simulink model "a4"  (R2018b)
settings: Solver=ode23tb  StartTime=0.0  StopTime=24*60*60  MaxStep=60  RelTol=1e-4
PreLoadFcn:
  | load('solar_load_data_24h.mat')
(part 1 of 2)
settings Model: Creator=alavi  LastModifiedBy=alavi
settings SolverCC: InitialStep=1e-4
settings SFSimCC: SimUseLocalCustomCode=off
settings RTWCC: RTWUseLocalCustomCode=off
settings CodeAppCC: StateflowObjectComments=on

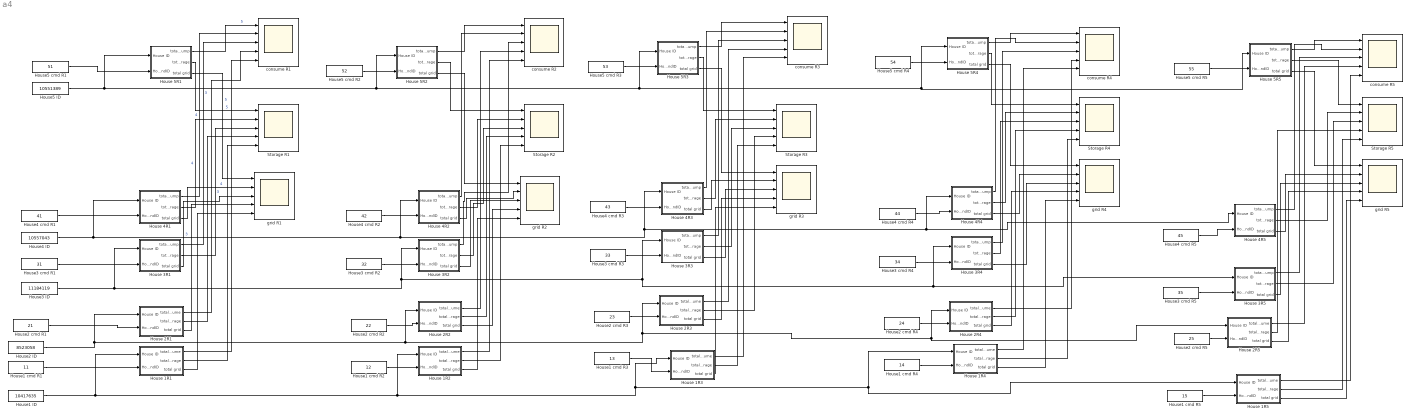
== system a4 ==
  House 1R1 : Subsystem
  House 1R2 : Subsystem
  House 1R3 : Subsystem
  House 1R4 : Subsystem
  House 1R5 : Subsystem
  House 2R1 : Subsystem
  House 2R2 : Subsystem
  House 2R3 : Subsystem
  House 2R4 : Subsystem
  House 2R5 : Subsystem
  House 3R1 : Subsystem
  House 3R2 : Subsystem
  House 3R3 : Subsystem
  House 3R4 : Subsystem
  House 3R5 : Subsystem
  House 4R1 : Subsystem
  House 4R2 : Subsystem
  House 4R3 : Subsystem
  House 4R4 : Subsystem
  House 4R5 : Subsystem
  House 5R1 : Subsystem
  House 5R2 : Subsystem
  House 5R3 : Subsystem
  House 5R4 : Subsystem
  House 5R5 : Subsystem
  House1 ID : Constant  Value=10417635
  House1 cmd R1 : Constant  Value=11
  House1 cmd R2 : Constant  Value=12
  House1 cmd R3 : Constant  Value=13
  House1 cmd R4 : Constant  Value=14
  House1 cmd R5 : Constant  Value=15
  House2 ID : Constant  Value=8523058
  House2 cmd R1 : Constant  Value=21
  House2 cmd R2 : Constant  Value=22
  House2 cmd R3 : Constant  Value=23
  House2 cmd R4 : Constant  Value=24
  House2 cmd R5 : Constant  Value=25
  House3 ID : Constant  Value=11184119
  House3 cmd R1 : Constant  Value=31
  House3 cmd R2 : Constant  Value=32
  House3 cmd R3 : Constant  Value=33
  House3 cmd R4 : Constant  Value=34
  House3 cmd R5 : Constant  Value=35
  House4 ID : Constant  Value=10557043
  House4 cmd R1 : Constant  Value=41
  House4 cmd R2 : Constant  Value=42
  House4 cmd R3 : Constant  Value=43
  House4 cmd R4 : Constant  Value=44
  House4 cmd R5 : Constant  Value=45
  House5 ID : Constant  Value=10551389
  House5 cmd R1 : Constant  Value=51
  House5 cmd R2 : Constant  Value=52
  House5 cmd R3 : Constant  Value=53
  House5 cmd R4 : Constant  Value=54
  House5 cmd R5 : Constant  Value=55
  "Storage R1 " : Scope  NumInputPorts=5
  Storage R{2..5} (4 alike) : Scope  NumInputPorts=5
  "consume R1 " : Scope  NumInputPorts=5
  consume R{2..5} (4 alike) : Scope  NumInputPorts=5
  "grid R1 " : Scope  NumInputPorts=5
  grid R{2..5} (4 alike) : Scope  NumInputPorts=5
  wires:
  House1 cmd R1/1 -> House 1R1/2(House CommandID)
  House2 cmd R1/1 -> House 2R1/2(House CommandID)
  House3 cmd R1/1 -> House 3R1/2(House CommandID)
  House4 cmd R1/1 -> House 4R1/2(House CommandID)
  House1 cmd R2/1 -> House 1R2/2(House CommandID)
  House2 cmd R2/1 -> House 2R2/2(House CommandID)
  House1 cmd R3/1 -> House 1R3/2(House CommandID)
  House2 cmd R3/1 -> House 2R3/2(House CommandID)
  House1 cmd R4/1 -> House 1R4/2(House CommandID)
  House2 cmd R4/1 -> House 2R4/2(House CommandID)
  House1 ID/1 -> House 1R2/1(House ID), House 1R3/1(House ID), House 1R5/1(House ID), House 1R4/1(House ID), House 1R1/1(House ID)
  House1 cmd R5/1 -> House 1R5/2(House CommandID)
  House4 cmd R2/1 -> House 4R2/2(House CommandID)
  House3 cmd R2/1 -> House 3R2/2(House CommandID)
  House4 cmd R3/1 -> House 4R3/2(House CommandID)
  House3 cmd R3/1 -> House 3R3/2(House CommandID)
  House4 cmd R4/1 -> House 4R4/2(House CommandID)
  House3 cmd R4/1 -> House 3R4/2(House CommandID)
  House4 cmd R5/1 -> House 4R5/2(House CommandID)
  House4 ID/1 -> House 4R1/1(House ID), House 4R2/1(House ID), House 4R3/1(House ID), House 4R5/1(House ID), House 4R4/1(House ID)
  House3 ID/1 -> House 3R1/1(House ID), House 3R2/1(House ID), House 3R3/1(House ID), House 3R5/1(House ID), House 3R4/1(House ID)
  House3 cmd R5/1 -> House 3R5/2(House CommandID)
  House5 cmd R2/1 -> House 5R2/2(House CommandID)
  House5 cmd R1/1 -> House 5R1/2(House CommandID)
  House5 ID/1 -> House 5R2/1(House ID), House 5R3/1(House ID), House 5R5/1(House ID), House 5R4/1(House ID), House 5R1/1(House ID)
  House5 cmd R3/1 -> House 5R3/2(House CommandID)
  House5 cmd R4/1 -> House 5R4/2(House CommandID)
  House5 cmd R5/1 -> House 5R5/2(House CommandID)
  House2 ID/1 -> House 2R2/1(House ID), House 2R3/1(House ID), House 2R5/1(House ID), House 2R4/1(House ID), House 2R1/1(House ID)
  House 5R1/1(total consump) -> "consume R1 "/1  "5"
  House 5R1/2(total storage) -> "Storage R1 "/1  "5"
  House 5R1/3(total grid) -> "grid R1 "/1  "5"
  House 5R2/1(total consump) -> consume R2/1
  House 5R2/2(total storage) -> Storage R2/1
  House 5R2/3(total grid) -> grid R2/1
  House 5R3/1(total consump) -> consume R3/1
  House 5R3/2(total storage) -> Storage R3/1
  House 5R3/3(total grid) -> grid R3/1
  House 5R4/1(total consump) -> consume R4/1
  House 5R4/2(total storage) -> Storage R4/1
  House 5R4/3(total grid) -> grid R4/1
  House 5R5/1(total consump) -> consume R5/1
  House 5R5/2(total storage) -> Storage R5/1
  House 5R5/3(total grid) -> grid R5/1
  House 4R1/1(total consump) -> "consume R1 "/2  "4"
  House 4R1/2(total storage) -> "Storage R1 "/2  "4"
  House 4R1/3(total grid) -> "grid R1 "/2  "4"
  House 3R1/1(total consump) -> "consume R1 "/3  "3"
  House 3R1/2(total storage) -> "Storage R1 "/3  "3"
  House 3R1/3(total grid) -> "grid R1 "/3  "3"
  House 4R2/1(total consump) -> consume R2/2
  House 4R2/2(total storage) -> Storage R2/2
  House 4R2/3(total grid) -> grid R2/2
  House 3R2/1(total consump) -> consume R2/3
  House 3R2/2(total storage) -> Storage R2/3
  House 3R2/3(total grid) -> grid R2/3
  House 4R3/1(total consump) -> consume R3/2
  House 4R3/2(total storage) -> Storage R3/2
  House 4R3/3(total grid) -> grid R3/2
  House 3R3/1(total consump) -> consume R3/3
  House 3R3/2(total storage) -> Storage R3/3
  House 3R3/3(total grid) -> grid R3/3
  House 4R4/1(total consump) -> consume R4/2
  House 4R4/2(total storage) -> Storage R4/2
  House 4R4/3(total grid) -> grid R4/2
  House 3R4/1(total consump) -> consume R4/3
  House 3R4/2(total storage) -> Storage R4/3
  House 3R4/3(total grid) -> grid R4/3
  House 4R5/1(total consump) -> consume R5/2
  House 4R5/2(total storage) -> Storage R5/2
  House 3R5/1(total consump) -> consume R5/3
  House 4R5/3(total grid) -> grid R5/2
  House 3R5/2(total storage) -> Storage R5/3
  House 3R5/3(total grid) -> grid R5/3
  House 2R1/1(total consume) -> "consume R1 "/4
  House 2R1/2(total storage) -> "Storage R1 "/4
  House 2R1/3(total grid) -> "grid R1 "/4
  House 2R2/1(total consume) -> consume R2/4
  House 2R2/2(total storage) -> Storage R2/4
  House 2R2/3(total grid) -> grid R2/4
  House 2R3/1(total consume) -> consume R3/4
  House 2R3/2(total storage) -> Storage R3/4
  House 2R3/3(total grid) -> grid R3/4
  House 2R4/1(total consume) -> consume R4/4
  House 2R4/2(total storage) -> Storage R4/4
  House 2R4/3(total grid) -> grid R4/4
  House 2R5/1(total consume) -> consume R5/4
  House 2R5/2(total storage) -> Storage R5/4
  House 2R5/3(total grid) -> grid R5/4
  House 1R1/1(total consume) -> "consume R1 "/5
  House 1R1/2(total storage) -> "Storage R1 "/5
  House 1R1/3(total grid) -> "grid R1 "/5
  House 1R2/1(total consume) -> consume R2/5
  House 1R2/2(total storage) -> Storage R2/5
  House 1R2/3(total grid) -> grid R2/5
  House 1R3/1(total consume) -> consume R3/5
  House 1R3/2(total storage) -> Storage R3/5
  House 1R3/3(total grid) -> grid R3/5
  House 1R4/1(total consume) -> consume R4/5
  House 1R4/2(total storage) -> Storage R4/5
  House 1R4/3(total grid) -> grid R4/5
  House 1R5/1(total consume) -> consume R5/5
  House 1R5/2(total storage) -> Storage R5/5
  House 1R5/3(total grid) -> grid R5/5
  House2 cmd R5/1 -> House 2R5/2(House CommandID)

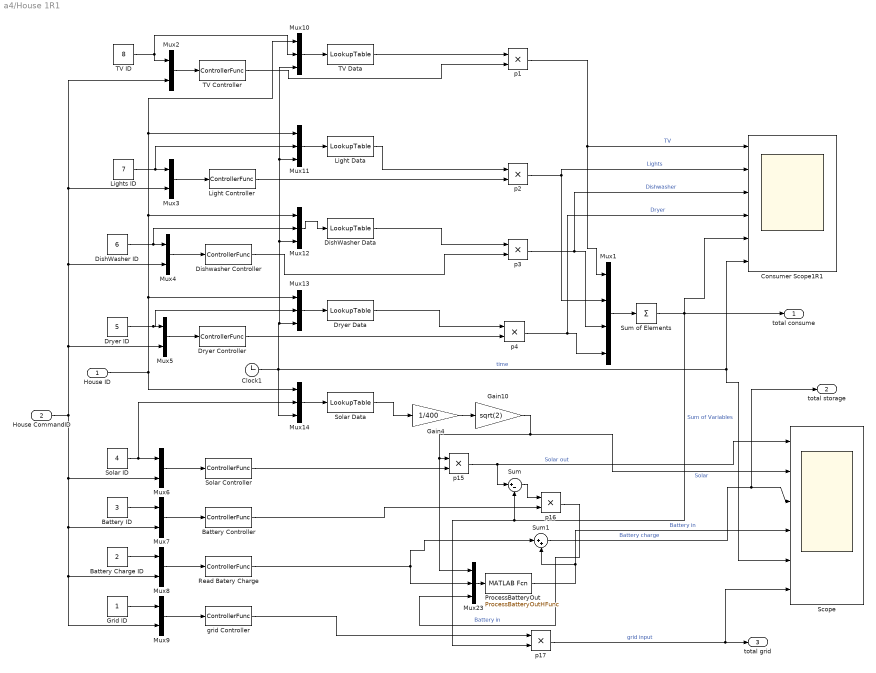
== system a4/House 1R1 ==
  House ID : Inport
  House CommandID : Inport  Port=2
  Battery Charge ID : Constant  Value=2
  Battery Controller : MATLABFcn  MATLABFcn=ControllerFunc  OutputSignalType=real
  Battery ID : Constant  Value=3
  Clock1 : Clock
  Consumer Scope1R1 : Scope  NumInputPorts=6
  DishWasher Data : MATLABFcn  MATLABFcn=LookupTable  OutputSignalType=real
  DishWasher ID : Constant  Value=6
  Dishwasher Controller : MATLABFcn  MATLABFcn=ControllerFunc  OutputSignalType=real
  Dryer Controller : MATLABFcn  MATLABFcn=ControllerFunc  OutputSignalType=real
  Dryer Data : MATLABFcn  MATLABFcn=LookupTable  OutputSignalType=real
  Dryer ID : Constant  Value=5
  Gain10 : Gain  Gain=sqrt(2)
  Gain4 : Gain  Gain=1/400
  Grid ID : Constant
  Light Controller : MATLABFcn  MATLABFcn=ControllerFunc  OutputSignalType=real
  Light Data : MATLABFcn  MATLABFcn=LookupTable  OutputSignalType=real
  Lights ID : Constant  Value=7
  Mux1 : Mux
  Mux{10..14,23} (6 alike) : Mux  Inputs=3
  Mux{2..9} (8 alike) : Mux  Inputs=2
  ProcessBatteryOut : MATLABFcn  MATLABFcn=ProcessBatteryOutHFunc  OutputSignalType=real
  Read Batery Charge : MATLABFcn  MATLABFcn=ControllerFunc  OutputSignalType=real
  Scope : Scope  NumInputPorts=6
  Solar Controller : MATLABFcn  MATLABFcn=ControllerFunc  OutputSignalType=real
  Solar Data : MATLABFcn  MATLABFcn=LookupTable  OutputSignalType=real
  Solar ID : Constant  Value=4
  Sum : Sum  Inputs=|+-
  Sum of Elements : Sum  Inputs=+
  Sum1 : Sum  Inputs=|++
  TV Controller : MATLABFcn  MATLABFcn=ControllerFunc  OutputSignalType=real
  TV Data : MATLABFcn  MATLABFcn=LookupTable  OutputSignalType=real
  TV ID : Constant  Value=8
  grid Controller : MATLABFcn  MATLABFcn=ControllerFunc  OutputSignalType=real
  p{1..4,15..17} (7 alike) : Product
  total consume : Outport
  total storage : Outport  Port=2
  total grid : Outport  Port=3
  wires:
  Clock1/1 -> Mux11/3, Mux10/3, Mux12/3, Mux13/3, Mux14/3, Scope/5, Consumer Scope1R1/6  "time"
  TV Data/1 -> p1/1
  Mux1/1 -> Sum of Elements/1
  p1/1 -> Consumer Scope1R1/1, Mux1/1  "TV"
  Sum of Elements/1 -> Consumer Scope1R1/5, total consume/1, p17/2, Sum/2  "Sum of Variables"
  p4/1 -> Consumer Scope1R1/4, Mux1/4  "Dryer"
  p2/1 -> Consumer Scope1R1/2, Mux1/2  "Lights"
  p3/1 -> Consumer Scope1R1/3, Mux1/3  "Dishwasher"
  Light Controller/1 -> p2/2
  Dishwasher Controller/1 -> p3/2
  Solar Data/1 -> Gain4/1
  Solar Controller/1 -> p15/2
  Gain10/1 -> Scope/2, Mux23/1, p15/1  "Solar"
  p15/1 -> Sum/1, Scope/1  "Solar out"
  Sum/1 -> p16/1
  Battery Controller/1 -> p16/2
  Sum1/1 -> total storage/1, Scope/3  "Battery charge"
  grid Controller/1 -> p17/1
  p17/1 -> Scope/6, total grid/1  "grid input"
  Read Batery Charge/1 -> Mux23/2, Sum1/1
  p16/1 -> Mux23/3  "Battery in"
  ProcessBatteryOut/1 -> Scope/4, Sum1/2  "Battery in"
  Light Data/1 -> p2/1
  DishWasher Data/1 -> p3/1
  Dryer Data/1 -> p4/1
  Dryer Controller/1 -> p4/2
  Gain4/1 -> Gain10/1
  TV ID/1 -> Mux2/1, Mux10/2
  House ID/1 -> Mux14/1, Mux10/1, Mux11/1, Mux12/1, Mux13/1
  Lights ID/1 -> Mux11/2, Mux3/1
  Mux3/1 -> Light Controller/1
  DishWasher ID/1 -> Mux12/2, Mux4/1
  Mux4/1 -> Dishwasher Controller/1
  Mux5/1 -> Dryer Controller/1
  Dryer ID/1 -> Mux13/2, Mux5/1
  Mux6/1 -> Solar Controller/1
  Solar ID/1 -> Mux14/2, Mux6/1
  Mux7/1 -> Battery Controller/1
  Mux8/1 -> Read Batery Charge/1
  Mux9/1 -> grid Controller/1
  Battery ID/1 -> Mux7/1
  Battery Charge ID/1 -> Mux8/1
  Grid ID/1 -> Mux9/1
  Mux10/1 -> TV Data/1
  Mux11/1 -> Light Data/1
  Mux12/1 -> DishWasher Data/1
  Mux13/1 -> Dryer Data/1
  Mux14/1 -> Solar Data/1
  TV Controller/1 -> p1/2
  Mux2/1 -> TV Controller/1
  House CommandID/1 -> Mux9/2, Mux8/2, Mux7/2, Mux6/2, Mux3/2, Mux2/2, Mux4/2, Mux5/2
  Mux23/1 -> ProcessBatteryOut/1

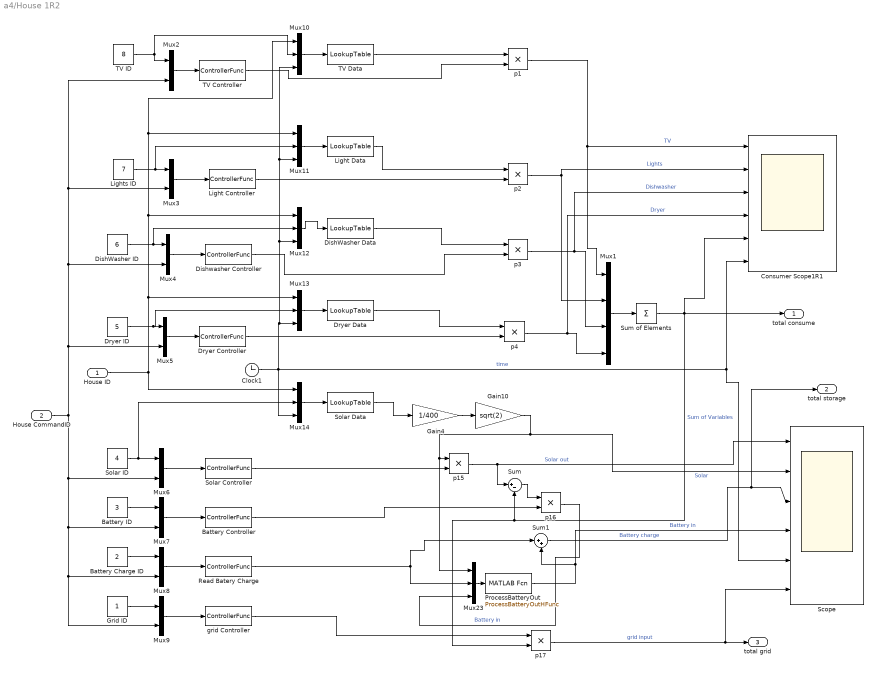
== system a4/House 1R2 ==
  House ID : Inport
  House CommandID : Inport  Port=2
  Battery Charge ID : Constant  Value=2
  Battery Controller : MATLABFcn  MATLABFcn=ControllerFunc  OutputSignalType=real
  Battery ID : Constant  Value=3
  Clock1 : Clock
  Consumer Scope1R1 : Scope  NumInputPorts=6
  DishWasher Data : MATLABFcn  MATLABFcn=LookupTable  OutputSignalType=real
  DishWasher ID : Constant  Value=6
  Dishwasher Controller : MATLABFcn  MATLABFcn=ControllerFunc  OutputSignalType=real
  Dryer Controller : MATLABFcn  MATLABFcn=ControllerFunc  OutputSignalType=real
  Dryer Data : MATLABFcn  MATLABFcn=LookupTable  OutputSignalType=real
  Dryer ID : Constant  Value=5
  Gain10 : Gain  Gain=sqrt(2)
  Gain4 : Gain  Gain=1/400
  Grid ID : Constant
  Light Controller : MATLABFcn  MATLABFcn=ControllerFunc  OutputSignalType=real
  Light Data : MATLABFcn  MATLABFcn=LookupTable  OutputSignalType=real
  Lights ID : Constant  Value=7
  Mux1 : Mux
  Mux{10..14,23} (6 alike) : Mux  Inputs=3
  Mux{2..9} (8 alike) : Mux  Inputs=2
  ProcessBatteryOut : MATLABFcn  MATLABFcn=ProcessBatteryOutHFunc  OutputSignalType=real
  Read Batery Charge : MATLABFcn  MATLABFcn=ControllerFunc  OutputSignalType=real
  Scope : Scope  NumInputPorts=6
  Solar Controller : MATLABFcn  MATLABFcn=ControllerFunc  OutputSignalType=real
  Solar Data : MATLABFcn  MATLABFcn=LookupTable  OutputSignalType=real
  Solar ID : Constant  Value=4
  Sum : Sum  Inputs=|+-
  Sum of Elements : Sum  Inputs=+
  Sum1 : Sum  Inputs=|++
  TV Controller : MATLABFcn  MATLABFcn=ControllerFunc  OutputSignalType=real
  TV Data : MATLABFcn  MATLABFcn=LookupTable  OutputSignalType=real
  TV ID : Constant  Value=8
  grid Controller : MATLABFcn  MATLABFcn=ControllerFunc  OutputSignalType=real
  p{1..4,15..17} (7 alike) : Product
  total consume : Outport
  total storage : Outport  Port=2
  total grid : Outport  Port=3
  wires:
  Mux23/1 -> ProcessBatteryOut/1
  House CommandID/1 -> Mux5/2, Mux4/2, Mux2/2, Mux3/2, Mux6/2, Mux7/2, Mux8/2, Mux9/2
  Mux2/1 -> TV Controller/1
  TV Controller/1 -> p1/2
  Mux14/1 -> Solar Data/1
  Mux13/1 -> Dryer Data/1
  Mux12/1 -> DishWasher Data/1
  Mux11/1 -> Light Data/1
  Mux10/1 -> TV Data/1
  Grid ID/1 -> Mux9/1
  Battery Charge ID/1 -> Mux8/1
  Battery ID/1 -> Mux7/1
  Mux9/1 -> grid Controller/1
  Mux8/1 -> Read Batery Charge/1
  Mux7/1 -> Battery Controller/1
  Solar ID/1 -> Mux6/1, Mux14/2
  Mux6/1 -> Solar Controller/1
  Dryer ID/1 -> Mux5/1, Mux13/2
  Mux5/1 -> Dryer Controller/1
  Mux4/1 -> Dishwasher Controller/1
  DishWasher ID/1 -> Mux4/1, Mux12/2
  Mux3/1 -> Light Controller/1
  Lights ID/1 -> Mux3/1, Mux11/2
  House ID/1 -> Mux13/1, Mux12/1, Mux11/1, Mux10/1, Mux14/1
  TV ID/1 -> Mux10/2, Mux2/1
  Gain4/1 -> Gain10/1
  Dryer Controller/1 -> p4/2
  Dryer Data/1 -> p4/1
  DishWasher Data/1 -> p3/1
  Light Data/1 -> p2/1
  ProcessBatteryOut/1 -> Sum1/2, Scope/4  "Battery in"
  p16/1 -> Mux23/3  "Battery in"
  Read Batery Charge/1 -> Sum1/1, Mux23/2
  p17/1 -> total grid/1, Scope/6  "grid input"
  grid Controller/1 -> p17/1
  Sum1/1 -> Scope/3, total storage/1  "Battery charge"
  Battery Controller/1 -> p16/2
  Sum/1 -> p16/1
  p15/1 -> Scope/1, Sum/1  "Solar out"
  Gain10/1 -> p15/1, Mux23/1, Scope/2  "Solar"
  Solar Controller/1 -> p15/2
  Solar Data/1 -> Gain4/1
  Dishwasher Controller/1 -> p3/2
  Light Controller/1 -> p2/2
  p3/1 -> Mux1/3, Consumer Scope1R1/3  "Dishwasher"
  p2/1 -> Mux1/2, Consumer Scope1R1/2  "Lights"
  p4/1 -> Mux1/4, Consumer Scope1R1/4  "Dryer"
  Sum of Elements/1 -> Sum/2, p17/2, total consume/1, Consumer Scope1R1/5  "Sum of Variables"
  p1/1 -> Mux1/1, Consumer Scope1R1/1  "TV"
  Mux1/1 -> Sum of Elements/1
  TV Data/1 -> p1/1
  Clock1/1 -> Consumer Scope1R1/6, Scope/5, Mux14/3, Mux13/3, Mux12/3, Mux10/3, Mux11/3  "time"

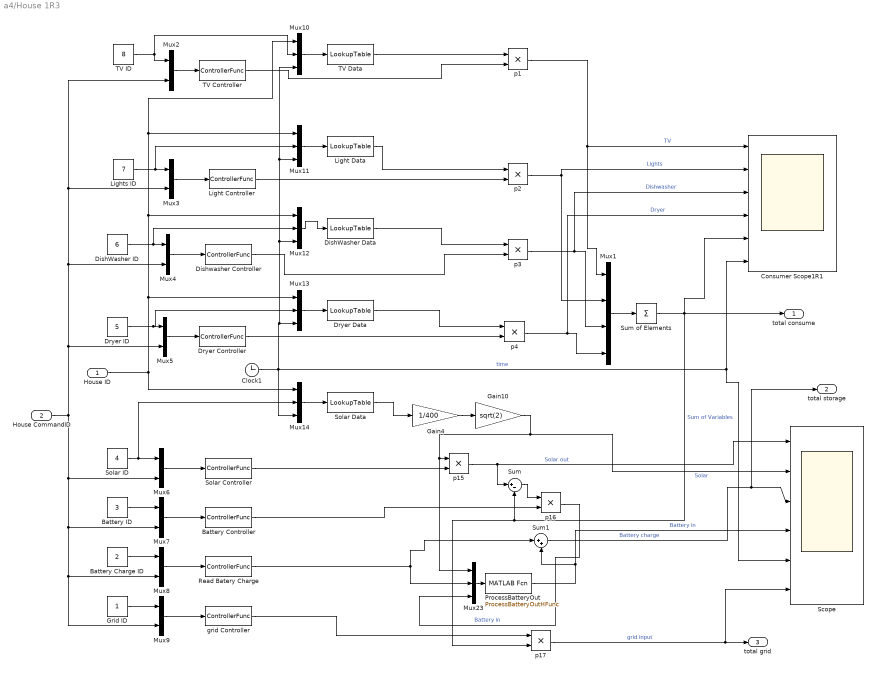
== system a4/House 1R3 ==
  House ID : Inport
  House CommandID : Inport  Port=2
  Battery Charge ID : Constant  Value=2
  Battery Controller : MATLABFcn  MATLABFcn=ControllerFunc  OutputSignalType=real
  Battery ID : Constant  Value=3
  Clock1 : Clock
  Consumer Scope1R1 : Scope  NumInputPorts=6
  DishWasher Data : MATLABFcn  MATLABFcn=LookupTable  OutputSignalType=real
  DishWasher ID : Constant  Value=6
  Dishwasher Controller : MATLABFcn  MATLABFcn=ControllerFunc  OutputSignalType=real
  Dryer Controller : MATLABFcn  MATLABFcn=ControllerFunc  OutputSignalType=real
  Dryer Data : MATLABFcn  MATLABFcn=LookupTable  OutputSignalType=real
  Dryer ID : Constant  Value=5
  Gain10 : Gain  Gain=sqrt(2)
  Gain4 : Gain  Gain=1/400
  Grid ID : Constant
  Light Controller : MATLABFcn  MATLABFcn=ControllerFunc  OutputSignalType=real
  Light Data : MATLABFcn  MATLABFcn=LookupTable  OutputSignalType=real
  Lights ID : Constant  Value=7
  Mux1 : Mux
  Mux{10..14,23} (6 alike) : Mux  Inputs=3
  Mux{2..9} (8 alike) : Mux  Inputs=2
  ProcessBatteryOut : MATLABFcn  MATLABFcn=ProcessBatteryOutHFunc  OutputSignalType=real
  Read Batery Charge : MATLABFcn  MATLABFcn=ControllerFunc  OutputSignalType=real
  Scope : Scope  NumInputPorts=6
  Solar Controller : MATLABFcn  MATLABFcn=ControllerFunc  OutputSignalType=real
  Solar Data : MATLABFcn  MATLABFcn=LookupTable  OutputSignalType=real
  Solar ID : Constant  Value=4
  Sum : Sum  Inputs=|+-
  Sum of Elements : Sum  Inputs=+
  Sum1 : Sum  Inputs=|++
  TV Controller : MATLABFcn  MATLABFcn=ControllerFunc  OutputSignalType=real
  TV Data : MATLABFcn  MATLABFcn=LookupTable  OutputSignalType=real
  TV ID : Constant  Value=8
  grid Controller : MATLABFcn  MATLABFcn=ControllerFunc  OutputSignalType=real
  p{1..4,15..17} (7 alike) : Product
  total consume : Outport
  total storage : Outport  Port=2
  total grid : Outport  Port=3
  wires:
  Clock1/1 -> Mux11/3, Mux10/3, Mux12/3, Mux13/3, Mux14/3, Scope/5, Consumer Scope1R1/6  "time"
  TV Data/1 -> p1/1
  Mux1/1 -> Sum of Elements/1
  p1/1 -> Consumer Scope1R1/1, Mux1/1  "TV"
  Sum of Elements/1 -> Consumer Scope1R1/5, total consume/1, p17/2, Sum/2  "Sum of Variables"
  p4/1 -> Consumer Scope1R1/4, Mux1/4  "Dryer"
  p2/1 -> Consumer Scope1R1/2, Mux1/2  "Lights"
  p3/1 -> Consumer Scope1R1/3, Mux1/3  "Dishwasher"
  Light Controller/1 -> p2/2
  Dishwasher Controller/1 -> p3/2
  Solar Data/1 -> Gain4/1
  Solar Controller/1 -> p15/2
  Gain10/1 -> Scope/2, Mux23/1, p15/1  "Solar"
  p15/1 -> Sum/1, Scope/1  "Solar out"
  Sum/1 -> p16/1
  Battery Controller/1 -> p16/2
  Sum1/1 -> total storage/1, Scope/3  "Battery charge"
  grid Controller/1 -> p17/1
  p17/1 -> Scope/6, total grid/1  "grid input"
  Read Batery Charge/1 -> Mux23/2, Sum1/1
  p16/1 -> Mux23/3  "Battery in"
  ProcessBatteryOut/1 -> Scope/4, Sum1/2  "Battery in"
  Light Data/1 -> p2/1
  DishWasher Data/1 -> p3/1
  Dryer Data/1 -> p4/1
  Dryer Controller/1 -> p4/2
  Gain4/1 -> Gain10/1
  TV ID/1 -> Mux2/1, Mux10/2
  House ID/1 -> Mux14/1, Mux10/1, Mux11/1, Mux12/1, Mux13/1
  Lights ID/1 -> Mux11/2, Mux3/1
  Mux3/1 -> Light Controller/1
  DishWasher ID/1 -> Mux12/2, Mux4/1
  Mux4/1 -> Dishwasher Controller/1
  Mux5/1 -> Dryer Controller/1
  Dryer ID/1 -> Mux13/2, Mux5/1
  Mux6/1 -> Solar Controller/1
  Solar ID/1 -> Mux14/2, Mux6/1
  Mux7/1 -> Battery Controller/1
  Mux8/1 -> Read Batery Charge/1
  Mux9/1 -> grid Controller/1
  Battery ID/1 -> Mux7/1
  Battery Charge ID/1 -> Mux8/1
  Grid ID/1 -> Mux9/1
  Mux10/1 -> TV Data/1
  Mux11/1 -> Light Data/1
  Mux12/1 -> DishWasher Data/1
  Mux13/1 -> Dryer Data/1
  Mux14/1 -> Solar Data/1
  TV Controller/1 -> p1/2
  Mux2/1 -> TV Controller/1
  House CommandID/1 -> Mux9/2, Mux8/2, Mux7/2, Mux6/2, Mux3/2, Mux2/2, Mux4/2, Mux5/2
  Mux23/1 -> ProcessBatteryOut/1

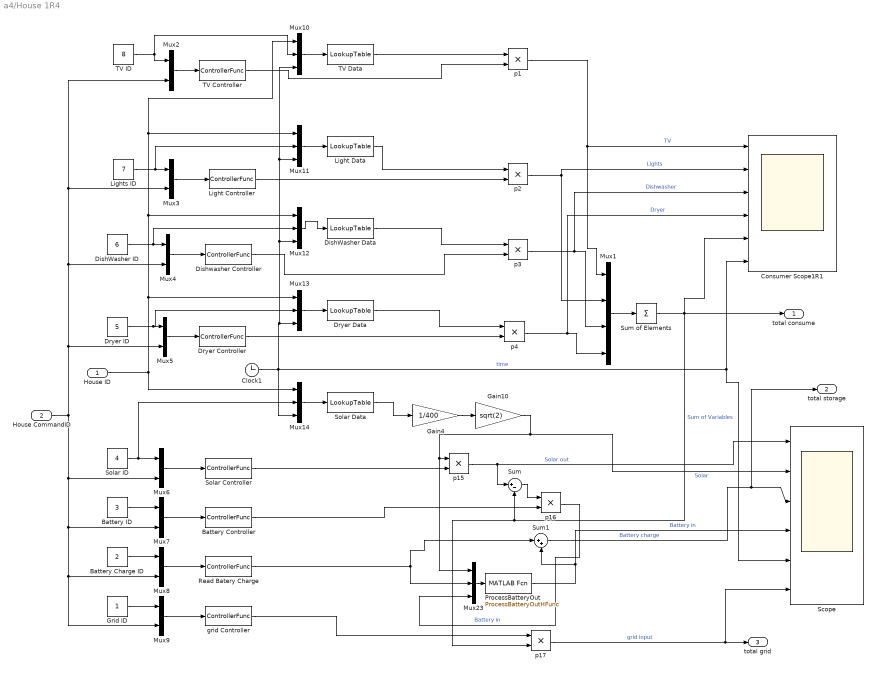
== system a4/House 1R4 ==
  House ID : Inport
  House CommandID : Inport  Port=2
  Battery Charge ID : Constant  Value=2
  Battery Controller : MATLABFcn  MATLABFcn=ControllerFunc  OutputSignalType=real
  Battery ID : Constant  Value=3
  Clock1 : Clock
  Consumer Scope1R1 : Scope  NumInputPorts=6
  DishWasher Data : MATLABFcn  MATLABFcn=LookupTable  OutputSignalType=real
  DishWasher ID : Constant  Value=6
  Dishwasher Controller : MATLABFcn  MATLABFcn=ControllerFunc  OutputSignalType=real
  Dryer Controller : MATLABFcn  MATLABFcn=ControllerFunc  OutputSignalType=real
  Dryer Data : MATLABFcn  MATLABFcn=LookupTable  OutputSignalType=real
  Dryer ID : Constant  Value=5
  Gain10 : Gain  Gain=sqrt(2)
  Gain4 : Gain  Gain=1/400
  Grid ID : Constant
  Light Controller : MATLABFcn  MATLABFcn=ControllerFunc  OutputSignalType=real
  Light Data : MATLABFcn  MATLABFcn=LookupTable  OutputSignalType=real
  Lights ID : Constant  Value=7
  Mux1 : Mux
  Mux{10..14,23} (6 alike) : Mux  Inputs=3
  Mux{2..9} (8 alike) : Mux  Inputs=2
  ProcessBatteryOut : MATLABFcn  MATLABFcn=ProcessBatteryOutHFunc  OutputSignalType=real
  Read Batery Charge : MATLABFcn  MATLABFcn=ControllerFunc  OutputSignalType=real
  Scope : Scope  NumInputPorts=6
  Solar Controller : MATLABFcn  MATLABFcn=ControllerFunc  OutputSignalType=real
  Solar Data : MATLABFcn  MATLABFcn=LookupTable  OutputSignalType=real
  Solar ID : Constant  Value=4
  Sum : Sum  Inputs=|+-
  Sum of Elements : Sum  Inputs=+
  Sum1 : Sum  Inputs=|++
  TV Controller : MATLABFcn  MATLABFcn=ControllerFunc  OutputSignalType=real
  TV Data : MATLABFcn  MATLABFcn=LookupTable  OutputSignalType=real
  TV ID : Constant  Value=8
  grid Controller : MATLABFcn  MATLABFcn=ControllerFunc  OutputSignalType=real
  p{1..4,15..17} (7 alike) : Product
  total consume : Outport
  total storage : Outport  Port=2
  total grid : Outport  Port=3
  wires:
  Mux23/1 -> ProcessBatteryOut/1
  House CommandID/1 -> Mux5/2, Mux4/2, Mux2/2, Mux3/2, Mux6/2, Mux7/2, Mux8/2, Mux9/2
  Mux2/1 -> TV Controller/1
  TV Controller/1 -> p1/2
  Mux14/1 -> Solar Data/1
  Mux13/1 -> Dryer Data/1
  Mux12/1 -> DishWasher Data/1
  Mux11/1 -> Light Data/1
  Mux10/1 -> TV Data/1
  Grid ID/1 -> Mux9/1
  Battery Charge ID/1 -> Mux8/1
  Battery ID/1 -> Mux7/1
  Mux9/1 -> grid Controller/1
  Mux8/1 -> Read Batery Charge/1
  Mux7/1 -> Battery Controller/1
  Solar ID/1 -> Mux6/1, Mux14/2
  Mux6/1 -> Solar Controller/1
  Dryer ID/1 -> Mux5/1, Mux13/2
  Mux5/1 -> Dryer Controller/1
  Mux4/1 -> Dishwasher Controller/1
  DishWasher ID/1 -> Mux4/1, Mux12/2
  Mux3/1 -> Light Controller/1
  Lights ID/1 -> Mux3/1, Mux11/2
  House ID/1 -> Mux13/1, Mux12/1, Mux11/1, Mux10/1, Mux14/1
  TV ID/1 -> Mux10/2, Mux2/1
  Gain4/1 -> Gain10/1
  Dryer Controller/1 -> p4/2
  Dryer Data/1 -> p4/1
  DishWasher Data/1 -> p3/1
  Light Data/1 -> p2/1
  ProcessBatteryOut/1 -> Sum1/2, Scope/4  "Battery in"
  p16/1 -> Mux23/3  "Battery in"
  Read Batery Charge/1 -> Sum1/1, Mux23/2
  p17/1 -> total grid/1, Scope/6  "grid input"
  grid Controller/1 -> p17/1
  Sum1/1 -> Scope/3, total storage/1  "Battery charge"
  Battery Controller/1 -> p16/2
  Sum/1 -> p16/1
  p15/1 -> Scope/1, Sum/1  "Solar out"
  Gain10/1 -> p15/1, Mux23/1, Scope/2  "Solar"
  Solar Controller/1 -> p15/2
  Solar Data/1 -> Gain4/1
  Dishwasher Controller/1 -> p3/2
  Light Controller/1 -> p2/2
  p3/1 -> Mux1/3, Consumer Scope1R1/3  "Dishwasher"
  p2/1 -> Mux1/2, Consumer Scope1R1/2  "Lights"
  p4/1 -> Mux1/4, Consumer Scope1R1/4  "Dryer"
  Sum of Elements/1 -> Sum/2, p17/2, total consume/1, Consumer Scope1R1/5  "Sum of Variables"
  p1/1 -> Mux1/1, Consumer Scope1R1/1  "TV"
  Mux1/1 -> Sum of Elements/1
  TV Data/1 -> p1/1
  Clock1/1 -> Consumer Scope1R1/6, Scope/5, Mux14/3, Mux13/3, Mux12/3, Mux10/3, Mux11/3  "time"

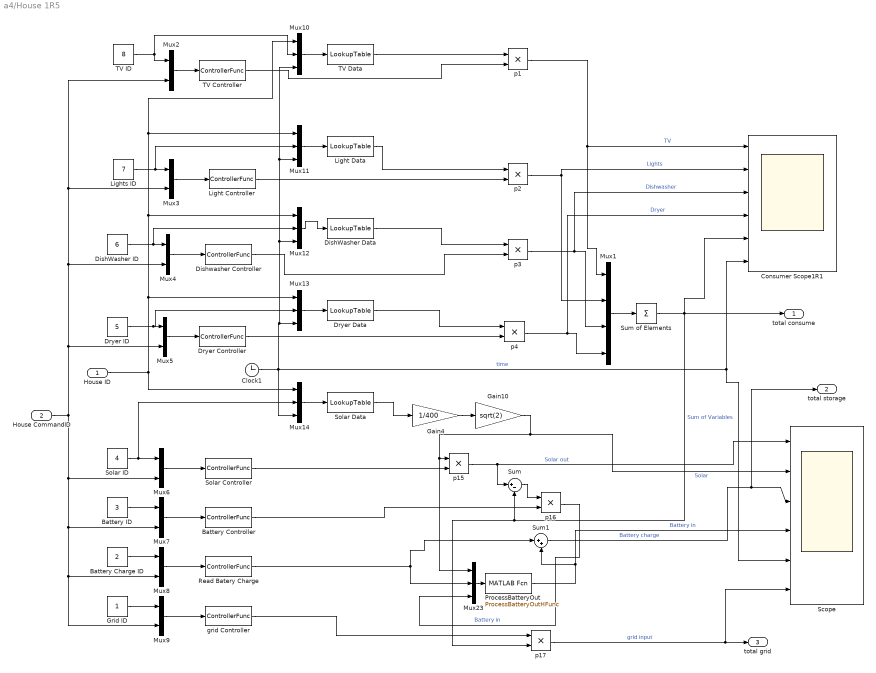
== system a4/House 1R5 ==
  House ID : Inport
  House CommandID : Inport  Port=2
  Battery Charge ID : Constant  Value=2
  Battery Controller : MATLABFcn  MATLABFcn=ControllerFunc  OutputSignalType=real
  Battery ID : Constant  Value=3
  Clock1 : Clock
  Consumer Scope1R1 : Scope  NumInputPorts=6
  DishWasher Data : MATLABFcn  MATLABFcn=LookupTable  OutputSignalType=real
  DishWasher ID : Constant  Value=6
  Dishwasher Controller : MATLABFcn  MATLABFcn=ControllerFunc  OutputSignalType=real
  Dryer Controller : MATLABFcn  MATLABFcn=ControllerFunc  OutputSignalType=real
  Dryer Data : MATLABFcn  MATLABFcn=LookupTable  OutputSignalType=real
  Dryer ID : Constant  Value=5
  Gain10 : Gain  Gain=sqrt(2)
  Gain4 : Gain  Gain=1/400
  Grid ID : Constant
  Light Controller : MATLABFcn  MATLABFcn=ControllerFunc  OutputSignalType=real
  Light Data : MATLABFcn  MATLABFcn=LookupTable  OutputSignalType=real
  Lights ID : Constant  Value=7
  Mux1 : Mux
  Mux{10..14,23} (6 alike) : Mux  Inputs=3
  Mux{2..9} (8 alike) : Mux  Inputs=2
  ProcessBatteryOut : MATLABFcn  MATLABFcn=ProcessBatteryOutHFunc  OutputSignalType=real
  Read Batery Charge : MATLABFcn  MATLABFcn=ControllerFunc  OutputSignalType=real
  Scope : Scope  NumInputPorts=6
  Solar Controller : MATLABFcn  MATLABFcn=ControllerFunc  OutputSignalType=real
  Solar Data : MATLABFcn  MATLABFcn=LookupTable  OutputSignalType=real
  Solar ID : Constant  Value=4
  Sum : Sum  Inputs=|+-
  Sum of Elements : Sum  Inputs=+
  Sum1 : Sum  Inputs=|++
  TV Controller : MATLABFcn  MATLABFcn=ControllerFunc  OutputSignalType=real
  TV Data : MATLABFcn  MATLABFcn=LookupTable  OutputSignalType=real
  TV ID : Constant  Value=8
  grid Controller : MATLABFcn  MATLABFcn=ControllerFunc  OutputSignalType=real
  p{1..4,15..17} (7 alike) : Product
  total consume : Outport
  total storage : Outport  Port=2
  total grid : Outport  Port=3
  wires:
  Clock1/1 -> Mux11/3, Mux10/3, Mux12/3, Mux13/3, Mux14/3, Scope/5, Consumer Scope1R1/6  "time"
  TV Data/1 -> p1/1
  Mux1/1 -> Sum of Elements/1
  p1/1 -> Consumer Scope1R1/1, Mux1/1  "TV"
  Sum of Elements/1 -> Consumer Scope1R1/5, total consume/1, p17/2, Sum/2  "Sum of Variables"
  p4/1 -> Consumer Scope1R1/4, Mux1/4  "Dryer"
  p2/1 -> Consumer Scope1R1/2, Mux1/2  "Lights"
  p3/1 -> Consumer Scope1R1/3, Mux1/3  "Dishwasher"
  Light Controller/1 -> p2/2
  Dishwasher Controller/1 -> p3/2
  Solar Data/1 -> Gain4/1
  Solar Controller/1 -> p15/2
  Gain10/1 -> Scope/2, Mux23/1, p15/1  "Solar"
  p15/1 -> Sum/1, Scope/1  "Solar out"
  Sum/1 -> p16/1
  Battery Controller/1 -> p16/2
  Sum1/1 -> total storage/1, Scope/3  "Battery charge"
  grid Controller/1 -> p17/1
  p17/1 -> Scope/6, total grid/1  "grid input"
  Read Batery Charge/1 -> Mux23/2, Sum1/1
  p16/1 -> Mux23/3  "Battery in"
  ProcessBatteryOut/1 -> Scope/4, Sum1/2  "Battery in"
  Light Data/1 -> p2/1
  DishWasher Data/1 -> p3/1
  Dryer Data/1 -> p4/1
  Dryer Controller/1 -> p4/2
  Gain4/1 -> Gain10/1
  TV ID/1 -> Mux2/1, Mux10/2
  House ID/1 -> Mux14/1, Mux10/1, Mux11/1, Mux12/1, Mux13/1
  Lights ID/1 -> Mux11/2, Mux3/1
  Mux3/1 -> Light Controller/1
  DishWasher ID/1 -> Mux12/2, Mux4/1
  Mux4/1 -> Dishwasher Controller/1
  Mux5/1 -> Dryer Controller/1
  Dryer ID/1 -> Mux13/2, Mux5/1
  Mux6/1 -> Solar Controller/1
  Solar ID/1 -> Mux14/2, Mux6/1
  Mux7/1 -> Battery Controller/1
  Mux8/1 -> Read Batery Charge/1
  Mux9/1 -> grid Controller/1
  Battery ID/1 -> Mux7/1
  Battery Charge ID/1 -> Mux8/1
  Grid ID/1 -> Mux9/1
  Mux10/1 -> TV Data/1
  Mux11/1 -> Light Data/1
  Mux12/1 -> DishWasher Data/1
  Mux13/1 -> Dryer Data/1
  Mux14/1 -> Solar Data/1
  TV Controller/1 -> p1/2
  Mux2/1 -> TV Controller/1
  House CommandID/1 -> Mux9/2, Mux8/2, Mux7/2, Mux6/2, Mux3/2, Mux2/2, Mux4/2, Mux5/2
  Mux23/1 -> ProcessBatteryOut/1

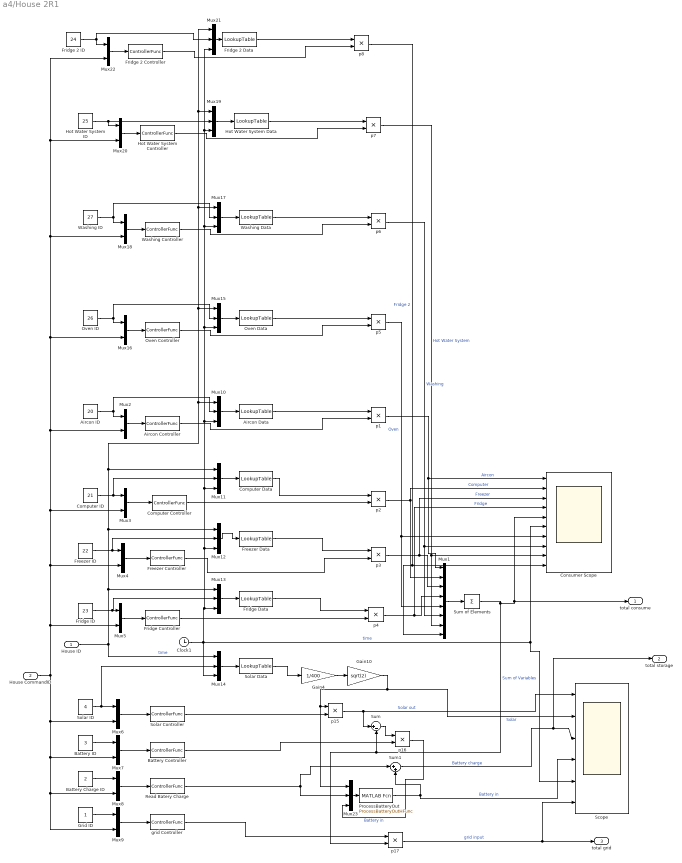
== system a4/House 2R1 ==
  House ID : Inport
  House CommandID : Inport  Port=2
  Aircon Controller : MATLABFcn  MATLABFcn=ControllerFunc  OutputSignalType=real
  Aircon Data : MATLABFcn  MATLABFcn=LookupTable  OutputSignalType=real
  Aircon ID : Constant  Value=20
  Battery Charge ID : Constant  Value=2
  Battery Controller : MATLABFcn  MATLABFcn=ControllerFunc  OutputSignalType=real
  Battery ID : Constant  Value=3
  Clock1 : Clock
  Computer Controller : MATLABFcn  MATLABFcn=ControllerFunc  OutputSignalType=real
  Computer Data : MATLABFcn  MATLABFcn=LookupTable  OutputSignalType=real
  Computer ID : Constant  Value=21
  Consumer Scope : Scope  NumInputPorts=10
  Freezer Controller : MATLABFcn  MATLABFcn=ControllerFunc  OutputSignalType=real
  Freezer Data : MATLABFcn  MATLABFcn=LookupTable  OutputSignalType=real
  Freezer ID : Constant  Value=22
  Fridge 2 Controller : MATLABFcn  MATLABFcn=ControllerFunc  OutputSignalType=real
  Fridge 2 Data : MATLABFcn  MATLABFcn=LookupTable  OutputSignalType=real
  Fridge 2 ID : Constant  Value=24
  Fridge Controller : MATLABFcn  MATLABFcn=ControllerFunc  OutputSignalType=real
  Fridge Data : MATLABFcn  MATLABFcn=LookupTable  OutputSignalType=real
  Fridge ID : Constant  Value=23
  Gain10 : Gain  Gain=sqrt(2)
  Gain4 : Gain  Gain=1/400
  Grid ID : Constant
  Hot Water System Controller : MATLABFcn  MATLABFcn=ControllerFunc  OutputSignalType=real
  Hot Water System Data : MATLABFcn  MATLABFcn=LookupTable  OutputSignalType=real
  Hot Water System ID : Constant  Value=25
  Mux1 : Mux  Inputs=8
  Mux{10..15,17,19,21,23} (10 alike) : Mux  Inputs=3
  Mux{2..9,16,18,20,22} (12 alike) : Mux  Inputs=2
  Oven Controller : MATLABFcn  MATLABFcn=ControllerFunc  OutputSignalType=real
  Oven Data : MATLABFcn  MATLABFcn=LookupTable  OutputSignalType=real
  Oven ID : Constant  Value=26
  ProcessBatteryOut : MATLABFcn  MATLABFcn=ProcessBatteryOutHFunc  OutputSignalType=real
  Read Batery Charge : MATLABFcn  MATLABFcn=ControllerFunc  OutputSignalType=real
  Scope : Scope  NumInputPorts=6
  Solar Controller : MATLABFcn  MATLABFcn=ControllerFunc  OutputSignalType=real
  Solar Data : MATLABFcn  MATLABFcn=LookupTable  OutputSignalType=real
  Solar ID : Constant  Value=4
  Sum : Sum  Inputs=|+-
  Sum of Elements : Sum  Inputs=+
  Sum1 : Sum  Inputs=|++
  Washing Controller : MATLABFcn  MATLABFcn=ControllerFunc  OutputSignalType=real
  Washing Data : MATLABFcn  MATLABFcn=LookupTable  OutputSignalType=real
  Washing ID : Constant  Value=27
  grid Controller : MATLABFcn  MATLABFcn=ControllerFunc  OutputSignalType=real
  p{1..8,15..17} (11 alike) : Product
  total consume : Outport
  total storage : Outport  Port=2
  total grid : Outport  Port=3
  wires:
  Clock1/1 -> Mux11/3, Mux21/3, Mux19/3, Mux17/3, Mux15/3, Mux10/3, Mux12/3, Mux13/3, Mux14/3, Scope/5, Consumer Scope/6  "time"
  Aircon Data/1 -> p1/1
  Mux1/1 -> Sum of Elements/1
  p1/1 -> Consumer Scope/1, Mux1/1  "Aircon"
  Sum of Elements/1 -> total consume/1, Consumer Scope/5, p17/2, Sum/2  "Sum of Variables"
  p4/1 -> Consumer Scope/4, Mux1/4  "Fridge"
  p2/1 -> Consumer Scope/2, Mux1/2  "Computer"
  p3/1 -> Consumer Scope/3, Mux1/3  "Freezer"
  Computer Controller/1 -> p2/2
  Freezer Controller/1 -> p3/2
  Solar Data/1 -> Gain4/1
  Solar Controller/1 -> p15/2
  Gain10/1 -> Scope/2, Mux23/1, p15/1  "Solar"
  p15/1 -> Sum/1, Scope/1  "Solar out"
  Sum/1 -> p16/1
  Battery Controller/1 -> p16/2
  Sum1/1 -> total storage/1, Scope/3  "Battery charge"
  grid Controller/1 -> p17/1
  p17/1 -> Scope/6, total grid/1  "grid input"
  Read Batery Charge/1 -> Mux23/2, Sum1/1
  p16/1 -> Mux23/3  "Battery in"
  ProcessBatteryOut/1 -> Scope/4, Sum1/2  "Battery in"
  Computer Data/1 -> p2/1
  Freezer Data/1 -> p3/1
  Fridge Data/1 -> p4/1
  Fridge Controller/1 -> p4/2
  Gain4/1 -> Gain10/1
  Aircon ID/1 -> Mux2/1, Mux10/2
  Computer ID/1 -> Mux11/2, Mux3/1
  Mux3/1 -> Computer Controller/1
  Freezer ID/1 -> Mux12/2, Mux4/1
  Mux4/1 -> Freezer Controller/1
  Mux5/1 -> Fridge Controller/1
  Fridge ID/1 -> Mux13/2, Mux5/1
  Mux6/1 -> Solar Controller/1
  Solar ID/1 -> Mux14/2, Mux6/1
  Mux7/1 -> Battery Controller/1
  Mux8/1 -> Read Batery Charge/1
  Mux9/1 -> grid Controller/1
  Battery ID/1 -> Mux7/1
  Battery Charge ID/1 -> Mux8/1
  Grid ID/1 -> Mux9/1
  Mux10/1 -> Aircon Data/1
  Mux11/1 -> Computer Data/1
  Mux12/1 -> Freezer Data/1
  Mux13/1 -> Fridge Data/1
  Mux14/1 -> Solar Data/1
  Aircon Controller/1 -> p1/2
  Mux2/1 -> Aircon Controller/1
  House CommandID/1 -> Mux9/2, Mux8/2, Mux7/2, Mux6/2, Mux3/2, Mux16/2, Mux20/2, Mux22/2, Mux18/2, Mux2/2, Mux4/2, Mux5/2
  Oven Data/1 -> p5/1
  Oven ID/1 -> Mux16/1, Mux15/2
  Mux15/1 -> Oven Data/1
  p5/1 -> Mux1/5, Consumer Scope/7  "Oven"
  Oven Controller/1 -> p5/2
  Washing Data/1 -> p6/1
  Washing ID/1 -> Mux18/1, Mux17/2
  Mux17/1 -> Washing Data/1
  p6/1 -> Mux1/6, Consumer Scope/8  "Washing"
  Washing Controller/1 -> p6/2
  Hot Water System Data/1 -> p7/1
  Hot Water System ID/1 -> Mux20/1, Mux19/2
  Mux19/1 -> Hot Water System Data/1
  p7/1 -> Mux1/7, Consumer Scope/9  "Hot Water System"
  Hot Water System Controller/1 -> p7/2
  Fridge 2 Data/1 -> p8/1
  Fridge 2 ID/1 -> Mux22/1, Mux21/2
  Mux21/1 -> Fridge 2 Data/1
  p8/1 -> Consumer Scope/10, Mux1/8  "Fridge 2"
  Fridge 2 Controller/1 -> p8/2
  House ID/1 -> Mux14/1, Mux21/1, Mux19/1, Mux17/1, Mux15/1, Mux10/1, Mux11/1, Mux12/1, Mux13/1  "time"
  Mux20/1 -> Hot Water System Controller/1
  Mux16/1 -> Oven Controller/1
  Mux18/1 -> Washing Controller/1
  Mux22/1 -> Fridge 2 Controller/1
  Mux23/1 -> ProcessBatteryOut/1

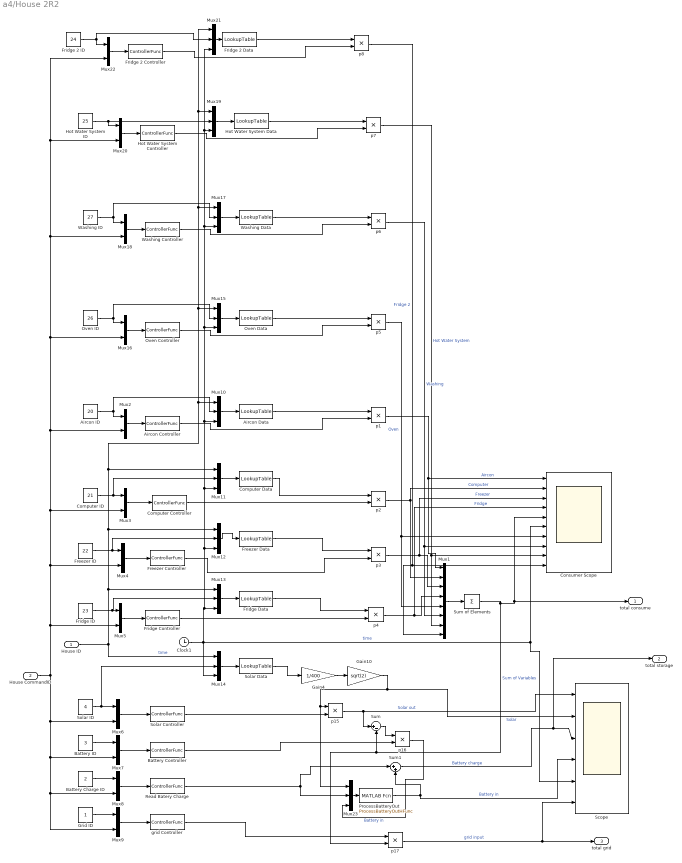
== system a4/House 2R2 ==
  House ID : Inport
  House CommandID : Inport  Port=2
  Aircon Controller : MATLABFcn  MATLABFcn=ControllerFunc  OutputSignalType=real
  Aircon Data : MATLABFcn  MATLABFcn=LookupTable  OutputSignalType=real
  Aircon ID : Constant  Value=20
  Battery Charge ID : Constant  Value=2
  Battery Controller : MATLABFcn  MATLABFcn=ControllerFunc  OutputSignalType=real
  Battery ID : Constant  Value=3
  Clock1 : Clock
  Computer Controller : MATLABFcn  MATLABFcn=ControllerFunc  OutputSignalType=real
  Computer Data : MATLABFcn  MATLABFcn=LookupTable  OutputSignalType=real
  Computer ID : Constant  Value=21
  Consumer Scope : Scope  NumInputPorts=10
  Freezer Controller : MATLABFcn  MATLABFcn=ControllerFunc  OutputSignalType=real
  Freezer Data : MATLABFcn  MATLABFcn=LookupTable  OutputSignalType=real
  Freezer ID : Constant  Value=22
  Fridge 2 Controller : MATLABFcn  MATLABFcn=ControllerFunc  OutputSignalType=real
  Fridge 2 Data : MATLABFcn  MATLABFcn=LookupTable  OutputSignalType=real
  Fridge 2 ID : Constant  Value=24
  Fridge Controller : MATLABFcn  MATLABFcn=ControllerFunc  OutputSignalType=real
  Fridge Data : MATLABFcn  MATLABFcn=LookupTable  OutputSignalType=real
  Fridge ID : Constant  Value=23
  Gain10 : Gain  Gain=sqrt(2)
  Gain4 : Gain  Gain=1/400
  Grid ID : Constant
  Hot Water System Controller : MATLABFcn  MATLABFcn=ControllerFunc  OutputSignalType=real
  Hot Water System Data : MATLABFcn  MATLABFcn=LookupTable  OutputSignalType=real
  Hot Water System ID : Constant  Value=25
  Mux1 : Mux  Inputs=8
  Mux{10..15,17,19,21,23} (10 alike) : Mux  Inputs=3
  Mux{2..9,16,18,20,22} (12 alike) : Mux  Inputs=2
  Oven Controller : MATLABFcn  MATLABFcn=ControllerFunc  OutputSignalType=real
  Oven Data : MATLABFcn  MATLABFcn=LookupTable  OutputSignalType=real
  Oven ID : Constant  Value=26
  ProcessBatteryOut : MATLABFcn  MATLABFcn=ProcessBatteryOutHFunc  OutputSignalType=real
  Read Batery Charge : MATLABFcn  MATLABFcn=ControllerFunc  OutputSignalType=real
  Scope : Scope  NumInputPorts=6
  Solar Controller : MATLABFcn  MATLABFcn=ControllerFunc  OutputSignalType=real
  Solar Data : MATLABFcn  MATLABFcn=LookupTable  OutputSignalType=real
  Solar ID : Constant  Value=4
  Sum : Sum  Inputs=|+-
  Sum of Elements : Sum  Inputs=+
  Sum1 : Sum  Inputs=|++
  Washing Controller : MATLABFcn  MATLABFcn=ControllerFunc  OutputSignalType=real
  Washing Data : MATLABFcn  MATLABFcn=LookupTable  OutputSignalType=real
  Washing ID : Constant  Value=27
  grid Controller : MATLABFcn  MATLABFcn=ControllerFunc  OutputSignalType=real
  p{1..8,15..17} (11 alike) : Product
  total consume : Outport
  total storage : Outport  Port=2
  total grid : Outport  Port=3
  wires:
  Mux23/1 -> ProcessBatteryOut/1
  Mux22/1 -> Fridge 2 Controller/1
  Mux18/1 -> Washing Controller/1
  Mux16/1 -> Oven Controller/1
  Mux20/1 -> Hot Water System Controller/1
  House ID/1 -> Mux13/1, Mux12/1, Mux11/1, Mux10/1, Mux15/1, Mux17/1, Mux19/1, Mux21/1, Mux14/1  "time"
  Fridge 2 Controller/1 -> p8/2
  p8/1 -> Mux1/8, Consumer Scope/10  "Fridge 2"
  Mux21/1 -> Fridge 2 Data/1
  Fridge 2 ID/1 -> Mux21/2, Mux22/1
  Fridge 2 Data/1 -> p8/1
  Hot Water System Controller/1 -> p7/2
  p7/1 -> Consumer Scope/9, Mux1/7  "Hot Water System"
  Mux19/1 -> Hot Water System Data/1
  Hot Water System ID/1 -> Mux19/2, Mux20/1
  Hot Water System Data/1 -> p7/1
  Washing Controller/1 -> p6/2
  p6/1 -> Consumer Scope/8, Mux1/6  "Washing"
  Mux17/1 -> Washing Data/1
  Washing ID/1 -> Mux17/2, Mux18/1
  Washing Data/1 -> p6/1
  Oven Controller/1 -> p5/2
  p5/1 -> Consumer Scope/7, Mux1/5  "Oven"
  Mux15/1 -> Oven Data/1
  Oven ID/1 -> Mux15/2, Mux16/1
  Oven Data/1 -> p5/1
  House CommandID/1 -> Mux5/2, Mux4/2, Mux2/2, Mux18/2, Mux22/2, Mux20/2, Mux16/2, Mux3/2, Mux6/2, Mux7/2, Mux8/2, Mux9/2
  Mux2/1 -> Aircon Controller/1
  Aircon Controller/1 -> p1/2
  Mux14/1 -> Solar Data/1
  Mux13/1 -> Fridge Data/1
  Mux12/1 -> Freezer Data/1
  Mux11/1 -> Computer Data/1
  Mux10/1 -> Aircon Data/1
  Grid ID/1 -> Mux9/1
  Battery Charge ID/1 -> Mux8/1
  Battery ID/1 -> Mux7/1
  Mux9/1 -> grid Controller/1
  Mux8/1 -> Read Batery Charge/1
  Mux7/1 -> Battery Controller/1
  Solar ID/1 -> Mux6/1, Mux14/2
  Mux6/1 -> Solar Controller/1
  Fridge ID/1 -> Mux5/1, Mux13/2
  Mux5/1 -> Fridge Controller/1
  Mux4/1 -> Freezer Controller/1
  Freezer ID/1 -> Mux4/1, Mux12/2
  Mux3/1 -> Computer Controller/1
  Computer ID/1 -> Mux3/1, Mux11/2
  Aircon ID/1 -> Mux10/2, Mux2/1
  Gain4/1 -> Gain10/1
  Fridge Controller/1 -> p4/2
  Fridge Data/1 -> p4/1
  Freezer Data/1 -> p3/1
  Computer Data/1 -> p2/1
  ProcessBatteryOut/1 -> Sum1/2, Scope/4  "Battery in"
  p16/1 -> Mux23/3  "Battery in"
  Read Batery Charge/1 -> Sum1/1, Mux23/2
  p17/1 -> total grid/1, Scope/6  "grid input"
  grid Controller/1 -> p17/1
  Sum1/1 -> Scope/3, total storage/1  "Battery charge"
  Battery Controller/1 -> p16/2
  Sum/1 -> p16/1
  p15/1 -> Scope/1, Sum/1  "Solar out"
  Gain10/1 -> p15/1, Mux23/1, Scope/2  "Solar"
  Solar Controller/1 -> p15/2
  Solar Data/1 -> Gain4/1
  Freezer Controller/1 -> p3/2
  Computer Controller/1 -> p2/2
  p3/1 -> Mux1/3, Consumer Scope/3  "Freezer"
  p2/1 -> Mux1/2, Consumer Scope/2  "Computer"
  p4/1 -> Mux1/4, Consumer Scope/4  "Fridge"
  Sum of Elements/1 -> Sum/2, p17/2, Consumer Scope/5, total consume/1  "Sum of Variables"
  p1/1 -> Mux1/1, Consumer Scope/1  "Aircon"
  Mux1/1 -> Sum of Elements/1
  Aircon Data/1 -> p1/1
  Clock1/1 -> Consumer Scope/6, Scope/5, Mux14/3, Mux13/3, Mux12/3, Mux10/3, Mux15/3, Mux17/3, Mux19/3, Mux21/3, Mux11/3  "time"

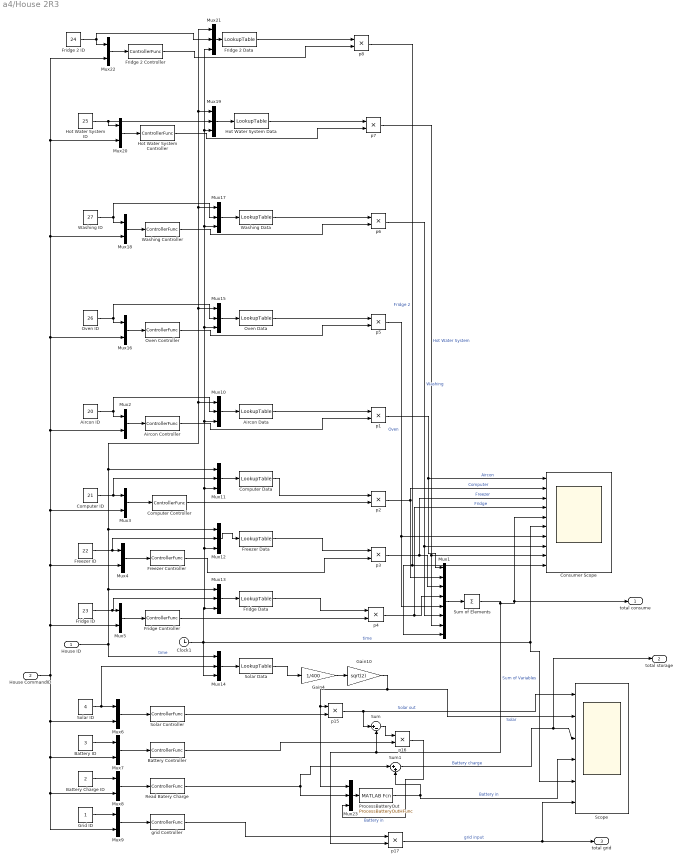
== system a4/House 2R3 ==
  House ID : Inport
  House CommandID : Inport  Port=2
  Aircon Controller : MATLABFcn  MATLABFcn=ControllerFunc  OutputSignalType=real
  Aircon Data : MATLABFcn  MATLABFcn=LookupTable  OutputSignalType=real
  Aircon ID : Constant  Value=20
  Battery Charge ID : Constant  Value=2
  Battery Controller : MATLABFcn  MATLABFcn=ControllerFunc  OutputSignalType=real
  Battery ID : Constant  Value=3
  Clock1 : Clock
  Computer Controller : MATLABFcn  MATLABFcn=ControllerFunc  OutputSignalType=real
  Computer Data : MATLABFcn  MATLABFcn=LookupTable  OutputSignalType=real
  Computer ID : Constant  Value=21
  Consumer Scope : Scope  NumInputPorts=10
  Freezer Controller : MATLABFcn  MATLABFcn=ControllerFunc  OutputSignalType=real
  Freezer Data : MATLABFcn  MATLABFcn=LookupTable  OutputSignalType=real
  Freezer ID : Constant  Value=22
  Fridge 2 Controller : MATLABFcn  MATLABFcn=ControllerFunc  OutputSignalType=real
  Fridge 2 Data : MATLABFcn  MATLABFcn=LookupTable  OutputSignalType=real
  Fridge 2 ID : Constant  Value=24
  Fridge Controller : MATLABFcn  MATLABFcn=ControllerFunc  OutputSignalType=real
  Fridge Data : MATLABFcn  MATLABFcn=LookupTable  OutputSignalType=real
  Fridge ID : Constant  Value=23
  Gain10 : Gain  Gain=sqrt(2)
  Gain4 : Gain  Gain=1/400
  Grid ID : Constant
  Hot Water System Controller : MATLABFcn  MATLABFcn=ControllerFunc  OutputSignalType=real
  Hot Water System Data : MATLABFcn  MATLABFcn=LookupTable  OutputSignalType=real
  Hot Water System ID : Constant  Value=25
  Mux1 : Mux  Inputs=8
  Mux{10..15,17,19,21,23} (10 alike) : Mux  Inputs=3
  Mux{2..9,16,18,20,22} (12 alike) : Mux  Inputs=2
  Oven Controller : MATLABFcn  MATLABFcn=ControllerFunc  OutputSignalType=real
  Oven Data : MATLABFcn  MATLABFcn=LookupTable  OutputSignalType=real
  Oven ID : Constant  Value=26
  ProcessBatteryOut : MATLABFcn  MATLABFcn=ProcessBatteryOutHFunc  OutputSignalType=real
  Read Batery Charge : MATLABFcn  MATLABFcn=ControllerFunc  OutputSignalType=real
  Scope : Scope  NumInputPorts=6
  Solar Controller : MATLABFcn  MATLABFcn=ControllerFunc  OutputSignalType=real
  Solar Data : MATLABFcn  MATLABFcn=LookupTable  OutputSignalType=real
  Solar ID : Constant  Value=4
  Sum : Sum  Inputs=|+-
  Sum of Elements : Sum  Inputs=+
  Sum1 : Sum  Inputs=|++
  Washing Controller : MATLABFcn  MATLABFcn=ControllerFunc  OutputSignalType=real
  Washing Data : MATLABFcn  MATLABFcn=LookupTable  OutputSignalType=real
  Washing ID : Constant  Value=27
  grid Controller : MATLABFcn  MATLABFcn=ControllerFunc  OutputSignalType=real
  p{1..8,15..17} (11 alike) : Product
  total consume : Outport
  total storage : Outport  Port=2
  total grid : Outport  Port=3
  wires:
  Clock1/1 -> Mux11/3, Mux21/3, Mux19/3, Mux17/3, Mux15/3, Mux10/3, Mux12/3, Mux13/3, Mux14/3, Scope/5, Consumer Scope/6  "time"
  Aircon Data/1 -> p1/1
  Mux1/1 -> Sum of Elements/1
  p1/1 -> Consumer Scope/1, Mux1/1  "Aircon"
  Sum of Elements/1 -> total consume/1, Consumer Scope/5, p17/2, Sum/2  "Sum of Variables"
  p4/1 -> Consumer Scope/4, Mux1/4  "Fridge"
  p2/1 -> Consumer Scope/2, Mux1/2  "Computer"
  p3/1 -> Consumer Scope/3, Mux1/3  "Freezer"
  Computer Controller/1 -> p2/2
  Freezer Controller/1 -> p3/2
  Solar Data/1 -> Gain4/1
  Solar Controller/1 -> p15/2
  Gain10/1 -> Scope/2, Mux23/1, p15/1  "Solar"
  p15/1 -> Sum/1, Scope/1  "Solar out"
  Sum/1 -> p16/1
  Battery Controller/1 -> p16/2
  Sum1/1 -> total storage/1, Scope/3  "Battery charge"
  grid Controller/1 -> p17/1
  p17/1 -> Scope/6, total grid/1  "grid input"
  Read Batery Charge/1 -> Mux23/2, Sum1/1
  p16/1 -> Mux23/3  "Battery in"
  ProcessBatteryOut/1 -> Scope/4, Sum1/2  "Battery in"
  Computer Data/1 -> p2/1
  Freezer Data/1 -> p3/1
  Fridge Data/1 -> p4/1
  Fridge Controller/1 -> p4/2
  Gain4/1 -> Gain10/1
  Aircon ID/1 -> Mux2/1, Mux10/2
  Computer ID/1 -> Mux11/2, Mux3/1
  Mux3/1 -> Computer Controller/1
  Freezer ID/1 -> Mux12/2, Mux4/1
  Mux4/1 -> Freezer Controller/1
  Mux5/1 -> Fridge Controller/1
  Fridge ID/1 -> Mux13/2, Mux5/1
  Mux6/1 -> Solar Controller/1
  Solar ID/1 -> Mux14/2, Mux6/1
  Mux7/1 -> Battery Controller/1
  Mux8/1 -> Read Batery Charge/1
  Mux9/1 -> grid Controller/1
  Battery ID/1 -> Mux7/1
  Battery Charge ID/1 -> Mux8/1
  Grid ID/1 -> Mux9/1
  Mux10/1 -> Aircon Data/1
  Mux11/1 -> Computer Data/1
  Mux12/1 -> Freezer Data/1
  Mux13/1 -> Fridge Data/1
  Mux14/1 -> Solar Data/1
  Aircon Controller/1 -> p1/2
  Mux2/1 -> Aircon Controller/1
  House CommandID/1 -> Mux9/2, Mux8/2, Mux7/2, Mux6/2, Mux3/2, Mux16/2, Mux20/2, Mux22/2, Mux18/2, Mux2/2, Mux4/2, Mux5/2
  Oven Data/1 -> p5/1
  Oven ID/1 -> Mux16/1, Mux15/2
  Mux15/1 -> Oven Data/1
  p5/1 -> Mux1/5, Consumer Scope/7  "Oven"
  Oven Controller/1 -> p5/2
  Washing Data/1 -> p6/1
  Washing ID/1 -> Mux18/1, Mux17/2
  Mux17/1 -> Washing Data/1
  p6/1 -> Mux1/6, Consumer Scope/8  "Washing"
  Washing Controller/1 -> p6/2
  Hot Water System Data/1 -> p7/1
  Hot Water System ID/1 -> Mux20/1, Mux19/2
  Mux19/1 -> Hot Water System Data/1
  p7/1 -> Mux1/7, Consumer Scope/9  "Hot Water System"
  Hot Water System Controller/1 -> p7/2
  Fridge 2 Data/1 -> p8/1
  Fridge 2 ID/1 -> Mux22/1, Mux21/2
  Mux21/1 -> Fridge 2 Data/1
  p8/1 -> Consumer Scope/10, Mux1/8  "Fridge 2"
  Fridge 2 Controller/1 -> p8/2
  House ID/1 -> Mux14/1, Mux21/1, Mux19/1, Mux17/1, Mux15/1, Mux10/1, Mux11/1, Mux12/1, Mux13/1  "time"
  Mux20/1 -> Hot Water System Controller/1
  Mux16/1 -> Oven Controller/1
  Mux18/1 -> Washing Controller/1
  Mux22/1 -> Fridge 2 Controller/1
  Mux23/1 -> ProcessBatteryOut/1

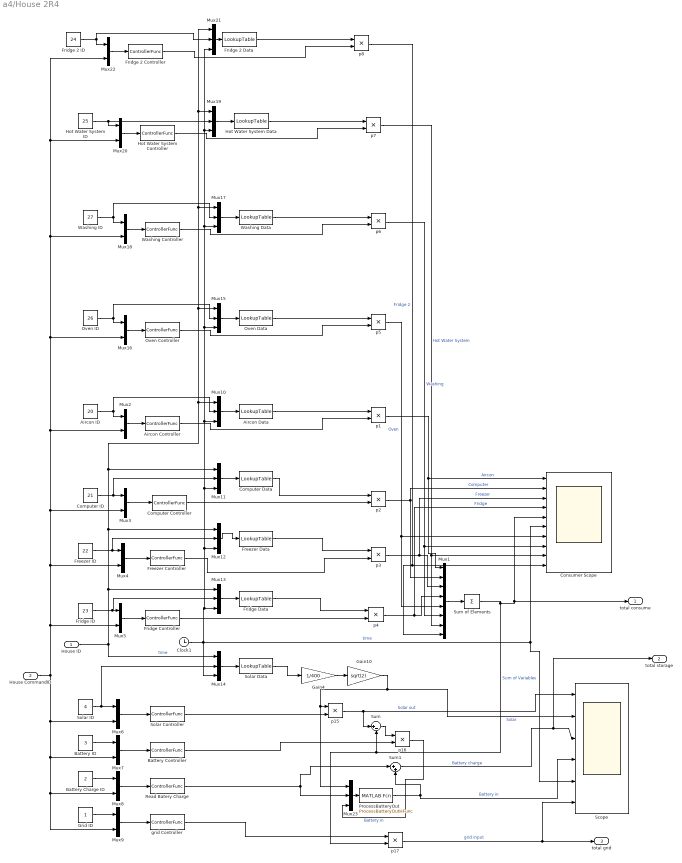
== system a4/House 2R4 ==
  House ID : Inport
  House CommandID : Inport  Port=2
  Aircon Controller : MATLABFcn  MATLABFcn=ControllerFunc  OutputSignalType=real
  Aircon Data : MATLABFcn  MATLABFcn=LookupTable  OutputSignalType=real
  Aircon ID : Constant  Value=20
  Battery Charge ID : Constant  Value=2
  Battery Controller : MATLABFcn  MATLABFcn=ControllerFunc  OutputSignalType=real
  Battery ID : Constant  Value=3
  Clock1 : Clock
  Computer Controller : MATLABFcn  MATLABFcn=ControllerFunc  OutputSignalType=real
  Computer Data : MATLABFcn  MATLABFcn=LookupTable  OutputSignalType=real
  Computer ID : Constant  Value=21
  Consumer Scope : Scope  NumInputPorts=10
  Freezer Controller : MATLABFcn  MATLABFcn=ControllerFunc  OutputSignalType=real
  Freezer Data : MATLABFcn  MATLABFcn=LookupTable  OutputSignalType=real
  Freezer ID : Constant  Value=22
  Fridge 2 Controller : MATLABFcn  MATLABFcn=ControllerFunc  OutputSignalType=real
  Fridge 2 Data : MATLABFcn  MATLABFcn=LookupTable  OutputSignalType=real
  Fridge 2 ID : Constant  Value=24
  Fridge Controller : MATLABFcn  MATLABFcn=ControllerFunc  OutputSignalType=real
  Fridge Data : MATLABFcn  MATLABFcn=LookupTable  OutputSignalType=real
  Fridge ID : Constant  Value=23
  Gain10 : Gain  Gain=sqrt(2)
  Gain4 : Gain  Gain=1/400
  Grid ID : Constant
  Hot Water System Controller : MATLABFcn  MATLABFcn=ControllerFunc  OutputSignalType=real
  Hot Water System Data : MATLABFcn  MATLABFcn=LookupTable  OutputSignalType=real
  Hot Water System ID : Constant  Value=25
  Mux1 : Mux  Inputs=8
  Mux{10..15,17,19,21,23} (10 alike) : Mux  Inputs=3
  Mux{2..9,16,18,20,22} (12 alike) : Mux  Inputs=2
  Oven Controller : MATLABFcn  MATLABFcn=ControllerFunc  OutputSignalType=real
  Oven Data : MATLABFcn  MATLABFcn=LookupTable  OutputSignalType=real
  Oven ID : Constant  Value=26
  ProcessBatteryOut : MATLABFcn  MATLABFcn=ProcessBatteryOutHFunc  OutputSignalType=real
  Read Batery Charge : MATLABFcn  MATLABFcn=ControllerFunc  OutputSignalType=real
  Scope : Scope  NumInputPorts=6
  Solar Controller : MATLABFcn  MATLABFcn=ControllerFunc  OutputSignalType=real
  Solar Data : MATLABFcn  MATLABFcn=LookupTable  OutputSignalType=real
  Solar ID : Constant  Value=4
  Sum : Sum  Inputs=|+-
  Sum of Elements : Sum  Inputs=+
  Sum1 : Sum  Inputs=|++
  Washing Controller : MATLABFcn  MATLABFcn=ControllerFunc  OutputSignalType=real
  Washing Data : MATLABFcn  MATLABFcn=LookupTable  OutputSignalType=real
  Washing ID : Constant  Value=27
  grid Controller : MATLABFcn  MATLABFcn=ControllerFunc  OutputSignalType=real
  p{1..8,15..17} (11 alike) : Product
  total consume : Outport
  total storage : Outport  Port=2
  total grid : Outport  Port=3
  wires:
  Mux23/1 -> ProcessBatteryOut/1
  Mux22/1 -> Fridge 2 Controller/1
  Mux18/1 -> Washing Controller/1
  Mux16/1 -> Oven Controller/1
  Mux20/1 -> Hot Water System Controller/1
  House ID/1 -> Mux13/1, Mux12/1, Mux11/1, Mux10/1, Mux15/1, Mux17/1, Mux19/1, Mux21/1, Mux14/1  "time"
  Fridge 2 Controller/1 -> p8/2
  p8/1 -> Mux1/8, Consumer Scope/10  "Fridge 2"
  Mux21/1 -> Fridge 2 Data/1
  Fridge 2 ID/1 -> Mux21/2, Mux22/1
  Fridge 2 Data/1 -> p8/1
  Hot Water System Controller/1 -> p7/2
  p7/1 -> Consumer Scope/9, Mux1/7  "Hot Water System"
  Mux19/1 -> Hot Water System Data/1
  Hot Water System ID/1 -> Mux19/2, Mux20/1
  Hot Water System Data/1 -> p7/1
  Washing Controller/1 -> p6/2
  p6/1 -> Consumer Scope/8, Mux1/6  "Washing"
  Mux17/1 -> Washing Data/1
  Washing ID/1 -> Mux17/2, Mux18/1
  Washing Data/1 -> p6/1
  Oven Controller/1 -> p5/2
  p5/1 -> Consumer Scope/7, Mux1/5  "Oven"
  Mux15/1 -> Oven Data/1
  Oven ID/1 -> Mux15/2, Mux16/1
  Oven Data/1 -> p5/1
  House CommandID/1 -> Mux5/2, Mux4/2, Mux2/2, Mux18/2, Mux22/2, Mux20/2, Mux16/2, Mux3/2, Mux6/2, Mux7/2, Mux8/2, Mux9/2
  Mux2/1 -> Aircon Controller/1
  Aircon Controller/1 -> p1/2
  Mux14/1 -> Solar Data/1
  Mux13/1 -> Fridge Data/1
  Mux12/1 -> Freezer Data/1
  Mux11/1 -> Computer Data/1
  Mux10/1 -> Aircon Data/1
  Grid ID/1 -> Mux9/1
  Battery Charge ID/1 -> Mux8/1
  Battery ID/1 -> Mux7/1
  Mux9/1 -> grid Controller/1
  Mux8/1 -> Read Batery Charge/1
  Mux7/1 -> Battery Controller/1
  Solar ID/1 -> Mux6/1, Mux14/2
  Mux6/1 -> Solar Controller/1
  Fridge ID/1 -> Mux5/1, Mux13/2
  Mux5/1 -> Fridge Controller/1
  Mux4/1 -> Freezer Controller/1
  Freezer ID/1 -> Mux4/1, Mux12/2
  Mux3/1 -> Computer Controller/1
  Computer ID/1 -> Mux3/1, Mux11/2
  Aircon ID/1 -> Mux10/2, Mux2/1
  Gain4/1 -> Gain10/1
  Fridge Controller/1 -> p4/2
  Fridge Data/1 -> p4/1
  Freezer Data/1 -> p3/1
  Computer Data/1 -> p2/1
  ProcessBatteryOut/1 -> Sum1/2, Scope/4  "Battery in"
  p16/1 -> Mux23/3  "Battery in"
  Read Batery Charge/1 -> Sum1/1, Mux23/2
  p17/1 -> total grid/1, Scope/6  "grid input"
  grid Controller/1 -> p17/1
  Sum1/1 -> Scope/3, total storage/1  "Battery charge"
  Battery Controller/1 -> p16/2
  Sum/1 -> p16/1
  p15/1 -> Scope/1, Sum/1  "Solar out"
  Gain10/1 -> p15/1, Mux23/1, Scope/2  "Solar"
  Solar Controller/1 -> p15/2
  Solar Data/1 -> Gain4/1
  Freezer Controller/1 -> p3/2
  Computer Controller/1 -> p2/2
  p3/1 -> Mux1/3, Consumer Scope/3  "Freezer"
  p2/1 -> Mux1/2, Consumer Scope/2  "Computer"
  p4/1 -> Mux1/4, Consumer Scope/4  "Fridge"
  Sum of Elements/1 -> Sum/2, p17/2, Consumer Scope/5, total consume/1  "Sum of Variables"
  p1/1 -> Mux1/1, Consumer Scope/1  "Aircon"
  Mux1/1 -> Sum of Elements/1
  Aircon Data/1 -> p1/1
  Clock1/1 -> Consumer Scope/6, Scope/5, Mux14/3, Mux13/3, Mux12/3, Mux10/3, Mux15/3, Mux17/3, Mux19/3, Mux21/3, Mux11/3  "time"
